simulink model "Simulinkasdasd"  (R2017a)
settings: Solver=ode45  StartTime=0.0  StopTime=1.5  RelTol=1e-3
undefined symbols (not defined in the file): B, Mn, psi, Rt, T, Un
libraries: powerlib x1
settings Model: Creator=user  LastModifiedBy=a
settings DataIOCC: LimitDataPoints=on  SaveFormat=Array  SignalLoggingSaveFormat=ModelDataLogs
settings OptimizationCC: BlockReduction=off  BooleanDataType=off  ExpressionDepthLimit=2147483647  LifeSpan=inf
settings DebuggingCC: SaveWithParameterizedLinksMsg=none  UnderspecifiedInitializationDetection=Classic  MergeDetectMultiDrivingBlocksExec=none  SignalResolutionControl=TryResolveAllWithWarning  MultiTaskDSMMsg=warning  MultiTaskCondExecSysMsg=none  StateNameClashWarn=warning  SFUnexpectedBacktrackingDiag=warning  SFNoUnconditionalDefaultTransitionDiag=warning  SFExecutionAtInitializationDiag=none
settings HardwareCC: ProdBitPerPointer=32  ProdBitPerSizeT=32  ProdBitPerPtrDiffT=32  ProdLargestAtomicFloat=None  ProdIntDivRoundTo=Undefined  ProdEndianess=Unspecified  ProdWordSize=32  ProdHWDeviceType=32-bit Generic  TargetUnknown=on
settings ModelReferenceCC: PropagateSignalLabelsOutOfModel=off
settings GRTTargetCC: TargetLangStandard=C89/C90 (ANSI)  GeneratePreprocessorConditionals=Disable all
settings ConfigComp: CovMetricSettings=dw  CovHtmlReporting=on  CovSaveCumulativeToWorkspaceVar=on  CovSaveSingleToWorkspaceVar=on  CovExternalEMLEnable=off

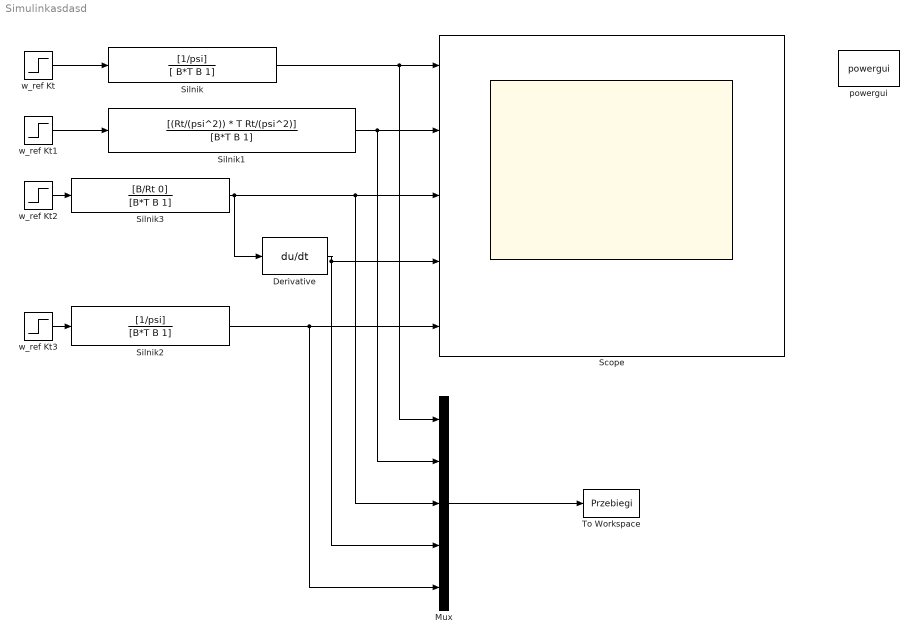
== system Simulinkasdasd ==
  Derivative : Derivative
  Mux : Mux  Inputs=5
  Scope : Scope  NumInputPorts=5
  Silnik : TransferFcn  Numerator=[1/psi]  Denominator=[ B*T B 1]
  Silnik1 : TransferFcn  Numerator=[(Rt/(psi^2)) * T Rt/(psi^2)]  Denominator=[B*T B 1]
  Silnik2 : TransferFcn  Numerator=[1/psi]  Denominator=[B*T B 1]
  Silnik3 : TransferFcn  Numerator=[B/Rt 0]  Denominator=[B*T B 1]
  To Workspace : ToWorkspace  VariableName=Przebiegi  SaveFormat=Structure With Time  SampleTime=-1
  powergui : powerlib/powergui  Priority=1  SimulationMode=Continuous  SampleTime=50e-6  frequency=60  Iterations=50  frequencyindice=60  Pbase=100e6  ErrMax=1e-4  UnitsV=kV  UnitsW=MW  buscounter=0  FunctionMessages=off  echomessages=off  EnableUseOfTLC=off  CurrentSourceSwitches=on  DisableSnubberDevices=off  DisableRonSwitches=off  DisableVfSwitches=off  DisplayEquations=off  SolverType=Tustin  Interpol=off  ExternalGateDelay=off  methode=off  Ts=100  x0status=blocks  SPID=off  SwTol=0  HookPort=off  RestoreLinks=warning  ResistiveCurrentMeasurement=off  Frange=[0:2:500]  Ylog=off  Xlog=on  ShowGrid=off  save=off  variable=ZData  structure=0  ZoomFFT=off  StartTime=0.0  cycles=1  DisplayStyle=1  fundamental=60  FreqAxis=off  MaxFrequency=1000  frequencyindicesteady=1  RmsSteady=1  display=off
  w_ref Kt : Step  Time=0  After=Un  SampleTime=0
  w_ref Kt1 : Step  Time=0  After=Mn  SampleTime=0
  w_ref Kt2 : Step  Time=0  After=Un  SampleTime=0
  w_ref Kt3 : Step  Time=0  After=Mn  SampleTime=0
  wires:
  Silnik/1 -> Mux/1, Scope/1
  Silnik1/1 -> Scope/2, Mux/2
  Silnik3/1 -> Derivative/1, Mux/3, Scope/3
  Silnik2/1 -> Mux/5, Scope/5
  w_ref Kt/1 -> Silnik/1
  w_ref Kt3/1 -> Silnik2/1
  w_ref Kt2/1 -> Silnik3/1
  w_ref Kt1/1 -> Silnik1/1
  Derivative/1 -> Mux/4, Scope/4
  Mux/1 -> To Workspace/1
